simulink model "BPPID"  (R2015a)
settings: Solver=ode4  StartTime=0.0  StopTime=100  FixedStep=0.01  RelTol=1e-3
settings Model: CovSFcnEnable=off  Creator=Administrator  LastModifiedBy=LAB425
settings SolverCC: AlgebraicLoopSolver=LineSearch
settings DataIOCC: SignalLoggingSaveFormat=ModelDataLogs
settings DebuggingCC: SolverPrmCheckMsg=warning  MultiTaskDSMMsg=warning  MultiTaskCondExecSysMsg=none

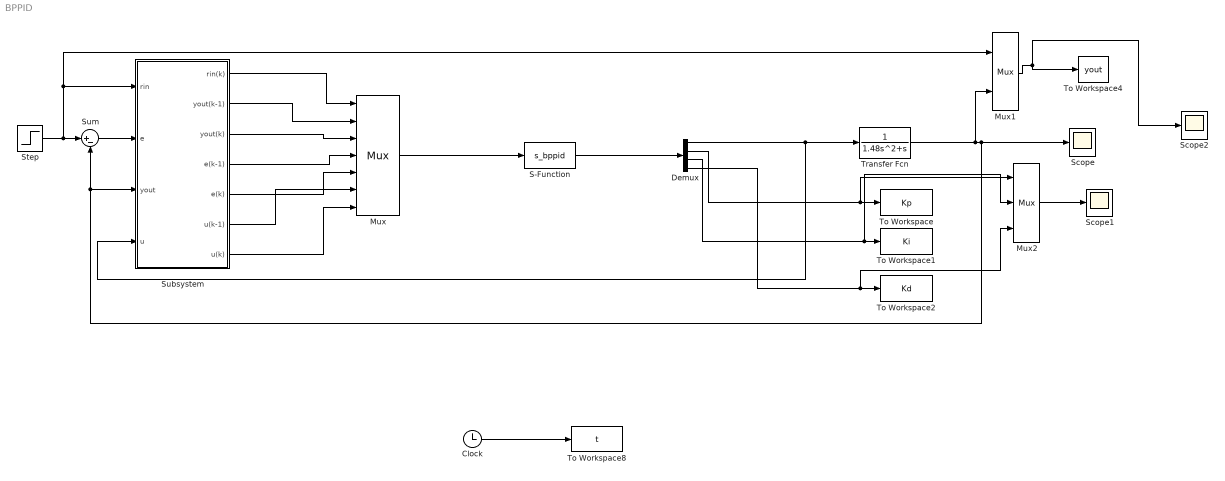
== system BPPID ==
  Clock : Clock
  Demux : Demux
  Mux : Mux  Inputs=7
  Mux1 : Mux  Inputs=2
  Mux2 : Mux  Inputs=3
  S-Function : S-Function  InitFcn=|  StartFcn=u=[1,0,0,1,1,0,0]  FunctionName=s_bppid
      | global wi;
      | wi=rand(5,3);
      | global wo;
      | wo=rand(3,5);
      | global wi_1;
      | global wi_2;
      | global wi_3;
      | global wo_1;
      | global wo_2;
      | global wo_3;
      | wi_1=wi;
      | wi_2=wi;
      | wi_3=wi;   
      | wo_1=wo;
      | wo_2=wo;
      | wo_3=wo;
      | global Kp;
      | Kp = 0;
      | global Ki;
      | Ki = 0;
      | global Kd;
      | Kd = 0;
  Scope : Scope
  Scope1 : Scope
  Scope2 : Scope
      settings: TimeRange=5  YMin=0.1  YMax=0.108  SaveName=ScopeData2
  Step : Step  Time=0  Before=1  SampleTime=0
  Subsystem : Subsystem
  Sum : Sum  Inputs=|+-  SampleTime=0
  To Workspace : ToWorkspace  VariableName=Kp  SampleTime=-1
  To Workspace1 : ToWorkspace  VariableName=Ki  SampleTime=-1
  To Workspace2 : ToWorkspace  VariableName=Kd  SampleTime=-1
  To Workspace4 : ToWorkspace  VariableName=yout  SampleTime=-1
  To Workspace8 : ToWorkspace  VariableName=t  SampleTime=-1
  Transfer Fcn : TransferFcn  Denominator=[1.48 1 0]
  wires:
  Subsystem/1(rin(k)) -> Mux/1
  Subsystem/2(yout(k-1)) -> Mux/2
  Subsystem/3(yout(k)) -> Mux/3
  Subsystem/4(e(k-1)) -> Mux/4
  Subsystem/5(e(k)) -> Mux/5
  Subsystem/6(u(k-1)) -> Mux/6
  Subsystem/7(u(k)) -> Mux/7
  Sum/1 -> Subsystem/2(e)
  Demux/2 -> Mux2/1, To Workspace/1
  Demux/3 -> Mux2/2, To Workspace1/1
  Demux/4 -> Mux2/3, To Workspace2/1
  Mux1/1 -> To Workspace4/1, Scope2/1
  Demux/1 -> Transfer Fcn/1, Subsystem/4(u)
  Mux/1 -> S-Function/1
  S-Function/1 -> Demux/1
  Clock/1 -> To Workspace8/1
  Transfer Fcn/1 -> Scope/1, Sum/2, Subsystem/3(yout), Mux1/2
  Step/1 -> Sum/1, Mux1/1, Subsystem/1(rin)
  Mux2/1 -> Scope1/1

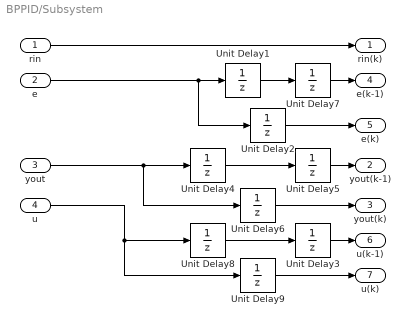
== system BPPID/Subsystem ==
  rin : Inport
  e : Inport  Port=2
  yout : Inport  Port=3
  u : Inport  Port=4
  Unit Delay{1..2,4,6..9} (7 alike) : UnitDelay  InitialCondition=1  SampleTime=0
  Unit Delay3 : UnitDelay  SampleTime=-1
  Unit Delay5 : UnitDelay  SampleTime=0
  rin(k) : Outport
  yout(k-1) : Outport  Port=2
  yout(k) : Outport  Port=3
  e(k-1) : Outport  Port=4
  e(k) : Outport  Port=5
  u(k-1) : Outport  Port=6
  u(k) : Outport  Port=7
  wires:
  rin/1 -> rin(k)/1
  Unit Delay3/1 -> u(k-1)/1
  Unit Delay5/1 -> yout(k-1)/1
  Unit Delay7/1 -> e(k-1)/1
  e/1 -> Unit Delay2/1, Unit Delay1/1
  yout/1 -> Unit Delay6/1, Unit Delay4/1
  u/1 -> Unit Delay9/1, Unit Delay8/1
  Unit Delay1/1 -> Unit Delay7/1
  Unit Delay2/1 -> e(k)/1
  Unit Delay4/1 -> Unit Delay5/1
  Unit Delay6/1 -> yout(k)/1
  Unit Delay9/1 -> u(k)/1
  Unit Delay8/1 -> Unit Delay3/1
